simulink model "PI_5_67"  (R2025a)
settings: Solver=VariableStepAuto  StartTime=0.0  StopTime=10.0  RelTol=1e-3
values from neighbouring files (symbols this model uses):
  alpha = a    (= 20.6731)    [Rocky_5_closed_loop_poles.m]    (also in pole5.m = a)
  beta = b    (= 0.001719)    [Rocky_5_closed_loop_poles.m]    (also in pole5.m = b)
  Ci = double(solutions.Ci)    [Rocky_5_closed_loop_poles.m]    (also in pole5.m = -2.7313)
  dist_duration = .1    (= 0.1)    [Rocky_5_closed_loop_poles.m]    (also in pole5.m)
  dist_magnitude = pi()/18    [Rocky_5_closed_loop_poles.m]    (also in pole5.m)
  dist_time = 1    [Rocky_5_closed_loop_poles.m]    (also in pole5.m)
  Ji = double(solutions.Ji)    [Rocky_5_closed_loop_poles.m]    (also in pole5.m = -105.9265)
  Jp = double(solutions.Jp)    [Rocky_5_closed_loop_poles.m]    (also in pole5.m = 247.1639)
  Ki = double(solutions.Ki)    [Rocky_5_closed_loop_poles.m]    (also in Rocky_closed_loop_poles_23.m; pole5.m = 16528)
  Kp = double(solutions.Kp)    [Rocky_5_closed_loop_poles.m]    (also in Rocky_closed_loop_poles_23.m; pole5.m = 3507.2)
  leff = l    (= 0.4452)    [Rocky_5_closed_loop_poles.m]    (also in pole5.m = l)
  omega_n = 4.6939    [Rocky_5_closed_loop_poles.m]    (also in pole5.m)
  theta_r = 0    [Rocky_5_closed_loop_poles.m]    (also in pole5.m)
libraries: slpidlib x1
settings Model: Creator=nbanse  LastModifiedBy=nbanse

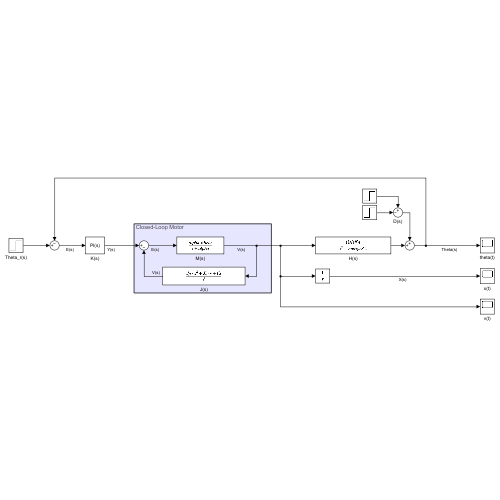
[thumbnail: Simulink's stored preview of the top-level diagram]
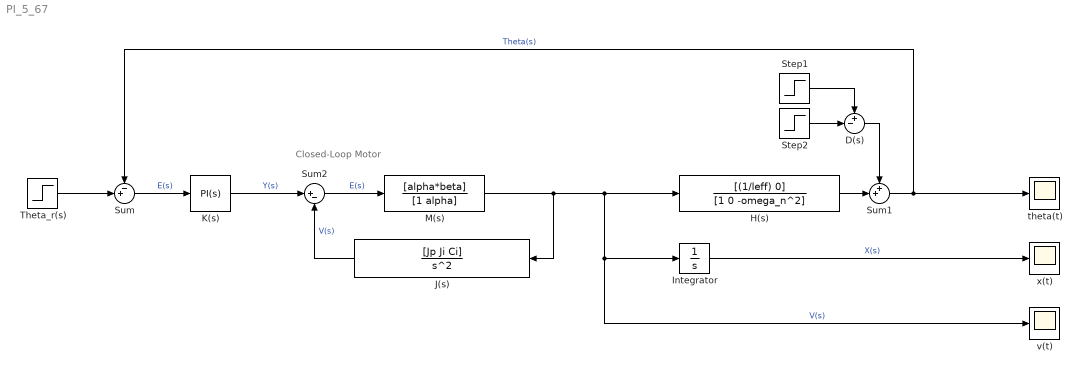
== system PI_5_67 ==
  note: Closed-Loop Motor
  D(s) : Sum  Inputs=+-|
  H(s) : TransferFcn  Numerator=[(1/leff) 0]  Denominator=[1 0 -omega_n^2]
  Integrator : Integrator
  J(s) : TransferFcn  Numerator=[Jp Ji Ci]  Denominator=[1 0 0]
  K(s) : slpidlib/PID Controller  Controller=PI  Form=Parallel  TimeDomain=Continuous-time  UseExternalTs=off  SampleTime=-1  IntegratorMethod=Forward Euler  FilterMethod=Forward Euler  ControllerParametersSource=internal  P=Kp  I=Ki  UseKiTs=off  D=0  UseExternalDerivativeSource=off  N=100  UseFilter=on  TunerSelectOption=Transfer Function Based (PID Tuner App)  InitialConditionSource=internal  InitialConditionForIntegrator=0  InitialConditionForFilter=0  DifferentiatorICPrevScaledInput=0  ExternalReset=none  TrackingMode=off  Kt=1  LimitOutput=off  SatLimitsSource=internal  UpperSaturationLimit=inf  LowerSaturationLimit=-inf  LinearizeAsGain=on  AntiWindupMode=none  Kb=1  LimitIntegrator=off  UpperIntegratorSaturationLimit=inf  LowerIntegratorSaturationLimit=-inf  POutMin=[]  POutMax=[]  IOutMin=[]  IOutMax=[]  DOutMin=[]  DOutMax=[]  NOutMin=[]  NOutMax=[]  SumOutMin=[]  SumOutMax=[]  SaturationOutMin=[]  SaturationOutMax=[]  PParamMin=[]  PParamMax=[]  IParamMin=[]  IParamMax=[]  DParamMin=[]  DParamMax=[]  NParamMin=[]  NParamMax=[]  KbParamMin=[]  KbParamMax=[]  KtParamMin=[]  KtParamMax=[]  KbOutMin=[]  KbOutMax=[]  KtOutMin=[]  KtOutMax=[]  IntegratorOutMin=[]  IntegratorOutMax=[]  FilterOutMin=[]  FilterOutMax=[]  SumI1OutMin=[]  SumI1OutMax=[]  SumI2OutMin=[]  SumI2OutMax=[]  SumI3OutMin=[]  SumI3OutMax=[]  SumI4OutMin=[]  SumI4OutMax=[]  SumDOutMin=[]  SumDOutMax=[]  DifferentiatorOutMin=[]  DifferentiatorOutMax=[]  FilterDiffOutCoefMin=[]  FilterDiffOutCoefMax=[]  ReciprocalOutMin=[]  ReciprocalOutMax=[]  SumDenOutMin=[]  SumDenOutMax=[]  SumNumOutMin=[]  SumNumOutMax=[]  DivideOutMin=[]  DivideOutMax=[]  UdiffTsProdOutMin=[]  UdiffTsProdOutMax=[]  NTsProdOutMin=[]  NTsProdOutMax=[]  UintegralTsProdOutMin=[]  UintegralTsProdOutMax=[]  UngainTsProdOutMin=[]  UngainTsProdOutMax=[]  ClampingZeroOutDataTypeStr=Inherit: Inherit via back propagation  ClampingZeroOutMin=[]  ClampingZeroOutMax=[]  FilterDenConstantOutDataTypeStr=Inherit: Inherit via back propagation  FilterDenConstantOutMin=[]  FilterDenConstantOutMax=[]  PCopyOutDataTypeStr=Inherit: Inherit via back propagation  PCopyOutMin=[]  PCopyOutMax=[]  NCopyOutDataTypeStr=Inherit: Inherit via back propagation  NCopyOutMin=[]  NCopyOutMax=[]  IntegratorContinuousStateAttributes=''  IntegratorStateMustResolveToSignalObject=off  IntegratorRTWStateStorageClass=Auto  FilterContinuousStateAttributes=''  FilterStateMustResolveToSignalObject=off  FilterRTWStateStorageClass=Auto  ParallelPVariant=InternalParameters  IdealPVariant=Disabled  IVariant=InternalParameters  DVariant=Disabled  IntegratorVariant=Continuous  SatVariant=Disabled  AWVariant=Passthrough  PCopyVariant=Disabled  TRVariant=Disabled  FdbkBlocksVariant=Forward  IdealPFdbkVariant=Disabled  SatFdbkVariant=Disabled  DerivativeFilterVariant=Disabled  NVariant=Disabled  NCopyVariant=Disabled_SignalSpec  FilterICVariant=Disabled  IntegratorICVariant=InternalICs  ExternalResetVariant=Disabled  TRSumVariant=Passthrough  SumFdbkVariant=Disabled  SumVariant=Sum_PI  TsampFilterVariant=InternalTs  TsampNgainVariant=Passthrough  TsampIntegralVariant=Disabled_SignalSpec  ExternalSaturationOutDataTypeStr=Inherit: Same as second input  DerivativeSourceVariant=Disabled  PreIntVariant=InternalPreInt
  M(s) : TransferFcn  Numerator=[alpha*beta]  Denominator=[1 alpha]
  Step1 : Step  Time=dist_time  After=dist_magnitude  SampleTime=0
  Step2 : Step  Time=dist_time+dist_duration  After=dist_magnitude  SampleTime=0
  Sum : Sum  Inputs=-+|
  Sum1 : Sum  Inputs=++|
  Sum2 : Sum  Inputs=|+-
  Theta_r(s) : Step  Time=0  After=theta_r  SampleTime=0
  theta(t) : Scope
      settings: ActiveDisplayYMinimum=-0.23282879296200232  ActiveDisplayYMaximum=0.2197953383284813
  v(t) : Scope
      settings: ActiveDisplayYMinimum=-1.0451283857472851  ActiveDisplayYMaximum=1.057707711864724  DataLoggingVariableName=ScopeData2
  x(t) : Scope
      settings: ActiveDisplayYMinimum=-0.11148407715549036  ActiveDisplayYMaximum=0.22663896509361078
  wires:
  H(s)/1 -> Sum1/2
  Step1/1 -> D(s)/1
  Step2/1 -> D(s)/2
  Sum/1 -> K(s)/1  "E(s)"
  D(s)/1 -> Sum1/1
  Sum1/1 -> Sum/1, theta(t)/1  "Theta(s)"
  Theta_r(s)/1 -> Sum/2
  Integrator/1 -> x(t)/1  "X(s)"
  K(s)/1 -> Sum2/1  "Y(s)"
  J(s)/1 -> Sum2/2  "V(s)"
  M(s)/1 -> v(t)/1, Integrator/1, H(s)/1, J(s)/1  "V(s)"
  Sum2/1 -> M(s)/1  "E(s)"
